simulink model "MODELO_HOGDKING_HUXELY_SBS"  (R2025b)
settings: Solver=ode45  StartTime=0  StopTime=2.5  MaxStep=1e-4  RelTol=1e-3
settings Model: Creator=fabri  LastModifiedBy=fabri

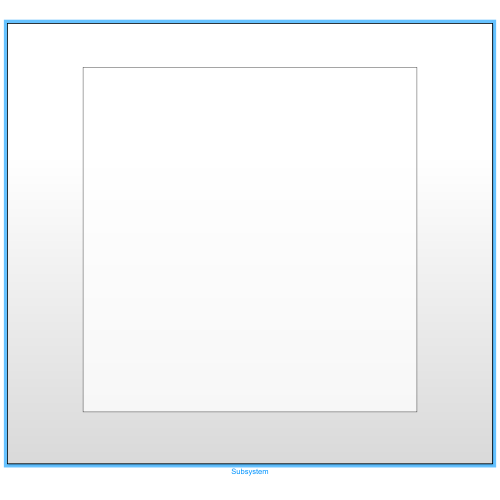
[thumbnail: Simulink's stored preview of the top-level diagram]
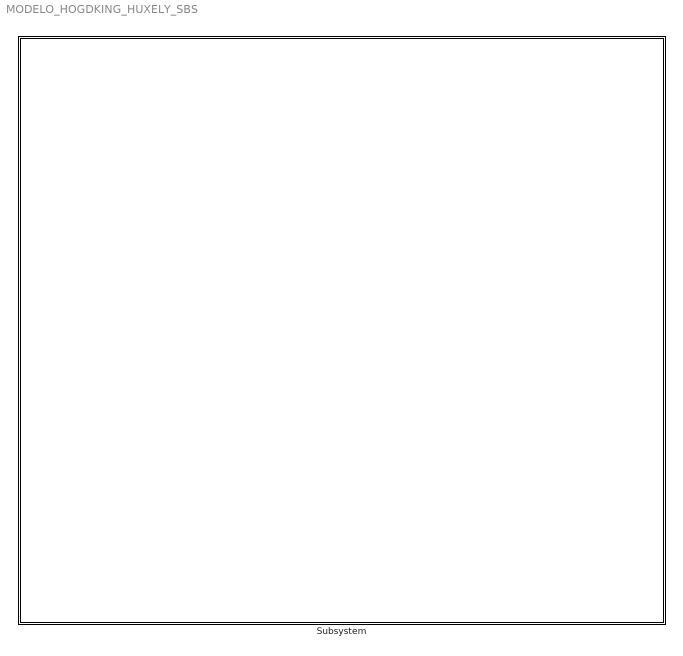
== system MODELO_HOGDKING_HUXELY_SBS ==
  Subsystem : Subsystem

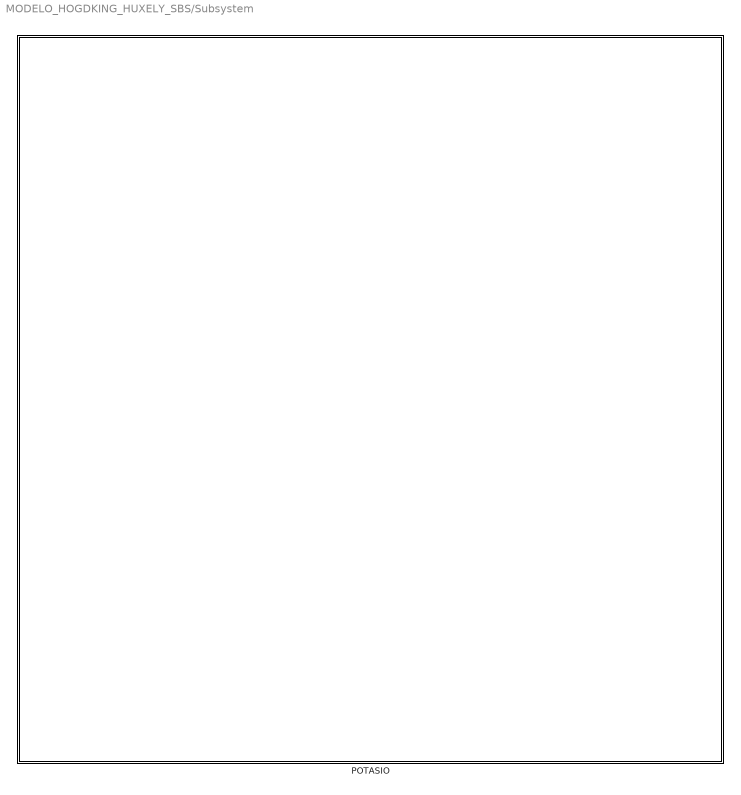
== system MODELO_HOGDKING_HUXELY_SBS/Subsystem ==
  POTASIO : Subsystem

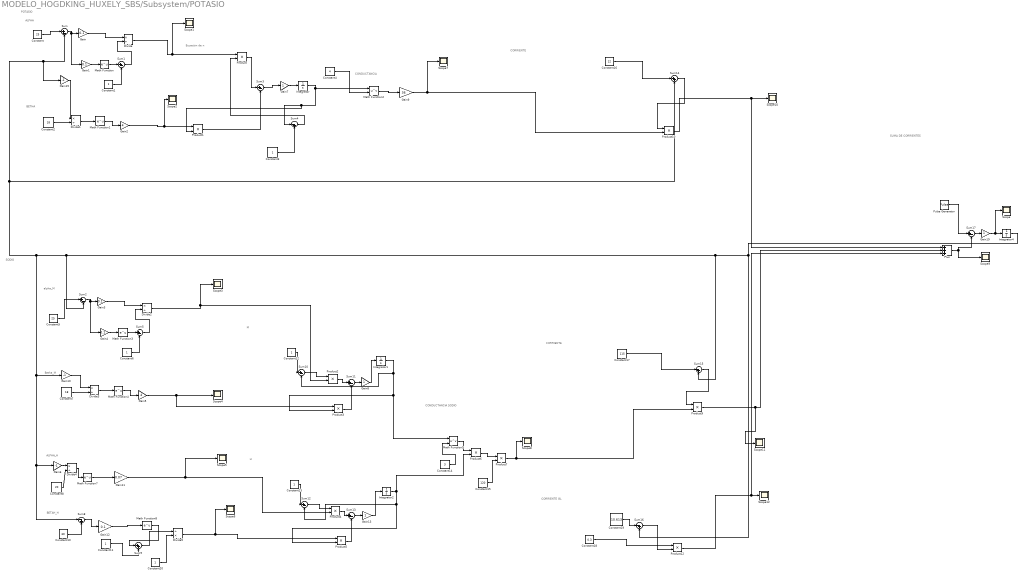
== system MODELO_HOGDKING_HUXELY_SBS/Subsystem/POTASIO ==
  note: CONDUCTANCIA SODIO
  note: M
  note: BETAH_H
  note: CONDUCTANCIA
  note: SODIO
  note: POTASIO
  note: Ecuación de n
  note: BETHA
  note: ALPHA
  note: alpha_M
  note: Betha_M
  note: ALPHA_H
  note: H
  note: CORRIENTE
  note: CORRIENTE
  note: SUMA DE CORRIENTES
  note: CORRIENTE GL
  Constant : Constant  Value=25
  Constant{1,3,6,11..13,20} (7 alike) : Constant
  Constant10 : Constant  Value=30
  Constant14 : Constant  Value=3
  Constant15 : Constant  Value=120
  Constant16 : Constant  Value=12
  Constant17 : Constant  Value=115
  Constant18 : Constant  Value=0.3
  Constant19 : Constant  Value=10.613
  Constant2 : Constant  Value=18
  Constant4 : Constant  Value=4
  Constant5 : Constant  Value=25
  Constant7 : Constant  Value=18
  Constant8 : Constant  Value=20
  Divide{,1..4} (5 alike) : Product  Inputs=*/
  Divide5 : Product  Inputs=/*
  Gain{,1,3..4,12} (5 alike) : Gain  Gain=0.1
  Gain10 : Gain  Gain=-1
  Gain11 : Gain  Gain=0.07
  Gain{7..8,13,19} (4 alike) : Gain
  Gain15 : Gain  Gain=-1
  Gain2 : Gain  Gain=4
  Gain5 : Gain  Gain=4
  Gain6 : Gain  Gain=-1
  Gain9 : Gain  Gain=36
  Integrator : Integrator  InitialCondition=0.317
  Integrator1 : Integrator  InitialCondition=0.05
  Integrator2 : Integrator  InitialCondition=0.6
  Integrator4 : Integrator  InitialCondition=60
  Math Function{,1,3..4,7..8} (6 alike) : Math
  Math Function2 : Math  Operator=pow
  Math Function9 : Math  Operator=pow
  Plus : Sum  Inputs=+++
  Product{,1..7,9..10,12} (11 alike) : Product
  Pulse Generator : DiscretePulseGenerator  PulseType=Time based  Amplitude=35  Period=50  PulseWidth=0.5  PhaseDelay=3
  Scope{,1..12} (13 alike) : Scope
      Scope settings: ActiveDisplayYMinimum=-95.1723618379546  ActiveDisplayYMaximum=59.6779141090574
      Scope1 settings: ActiveDisplayYMinimum=-0.17507037705461403  ActiveDisplayYMaximum=4.8064923190728459
      Scope10 settings: ActiveDisplayYMinimum=-182.23339181248534  ActiveDisplayYMaximum=1699.0889245773781  DataLoggingVariableName=ScopeData10
      Scope11 settings: ActiveDisplayYMinimum=-1  ActiveDisplayYMaximum=1  DataLoggingVariableName=ScopeData11
      Scope12 settings: ActiveDisplayYMinimum=-1  ActiveDisplayYMaximum=1  DataLoggingVariableName=ScopeData12
      Scope2 settings: ActiveDisplayYMinimum=-0.1237591277053367  ActiveDisplayYMaximum=2.0332343992823678  DataLoggingVariableName=ScopeData2
      Scope3 settings: ActiveDisplayYMinimum=-1  ActiveDisplayYMaximum=1  DataLoggingVariableName=ScopeData3
      Scope4 settings: ActiveDisplayYMinimum=-1  ActiveDisplayYMaximum=1  DataLoggingVariableName=ScopeData4
      Scope5 settings: ActiveDisplayYMinimum=-1  ActiveDisplayYMaximum=1  DataLoggingVariableName=ScopeData5
      Scope6 settings: ActiveDisplayYMinimum=-1  ActiveDisplayYMaximum=1  DataLoggingVariableName=ScopeData6
      Scope7 settings: ActiveDisplayYMinimum=-1  ActiveDisplayYMaximum=1  DataLoggingVariableName=ScopeData7
      Scope8 settings: ActiveDisplayYMinimum=-3.1594248054177867  ActiveDisplayYMaximum=28.524823248760089  DataLoggingVariableName=ScopeData8
      Scope9 settings: ActiveDisplayYMinimum=-1  ActiveDisplayYMaximum=1  DataLoggingVariableName=ScopeData9
  Sum{,1..3,5,10..13,17} (10 alike) : Sum  Inputs=|+-
  Sum14 : Sum  Inputs=|++
  Sum{4,8,15..16} (4 alike) : Sum  Inputs=|-+
  Sum9 : Sum  Inputs=|++
  wires:
  Constant/1 -> Sum/1
  Sum1/1 -> Divide/2
  Divide1/1 -> Math Function1/1
  Math Function/1 -> Sum1/1
  Sum/1 -> Gain1/1, Gain/1
  Constant2/1 -> Divide1/2
  Math Function1/1 -> Gain2/1
  Gain1/1 -> Math Function/1
  Constant1/1 -> Sum1/2
  Gain/1 -> Divide/1
  Product/1 -> Sum3/1
  Product1/1 -> Sum3/2
  Sum3/1 -> Gain7/1
  Integrator/1 -> Product1/2, Sum4/1, Math Function2/1
  Constant3/1 -> Sum4/2
  Sum4/1 -> Product/2
  Constant4/1 -> Math Function2/2
  Math Function4/1 -> Gain5/1
  Sum2/1 -> Gain4/1, Gain3/1
  Constant6/1 -> Sum5/2
  Constant7/1 -> Divide3/2
  Gain3/1 -> Divide2/1
  Divide3/1 -> Math Function4/1
  Gain4/1 -> Math Function3/1
  Constant5/1 -> Sum2/1
  Math Function3/1 -> Sum5/1
  Sum5/1 -> Divide2/2
  Math Function2/1 -> Gain9/1
  Math Function7/1 -> Gain11/1
  Constant10/1 -> Sum8/2
  Sum8/1 -> Gain12/1
  Constant11/1 -> Sum9/2
  Integrator1/1 -> Sum10/2, Math Function9/1, Product3/2
  Constant12/1 -> Sum10/1
  Sum10/1 -> Product2/1
  Product2/1 -> Sum11/1
  Product3/1 -> Sum11/2
  Sum11/1 -> Gain8/1
  Sum13/1 -> Gain13/1
  Sum12/1 -> Product4/1
  Divide5/1 -> Scope6/1, Product5/1
  Constant13/1 -> Sum12/1
  Product4/1 -> Sum13/1
  Product5/1 -> Sum13/2
  Integrator2/1 -> Sum12/2, Product5/2, Product6/2
  Constant14/1 -> Math Function9/2
  Math Function9/1 -> Product6/1
  Product6/1 -> Product7/1
  Constant15/1 -> Product7/2
  Product7/1 -> Scope8/1, Product9/2
  Constant16/1 -> Sum14/1
  Sum14/1 -> Product10/1
  Constant17/1 -> Sum15/1
  Constant18/1 -> Product12/1
  Constant19/1 -> Sum16/1
  Sum16/1 -> Product12/2
  Plus/1 -> Sum17/2, Scope9/1
  Constant20/1 -> Divide5/2
  Math Function8/1 -> Sum9/1
  Sum9/1 -> Divide5/1
  Gain12/1 -> Math Function8/1
  Gain9/1 -> Scope7/1, Product10/2
  Sum15/1 -> Product9/1
  Product12/1 -> Plus/3, Scope12/1
  Product10/1 -> Plus/1, Scope10/1
  Pulse Generator/1 -> Sum17/1
  Sum17/1 -> Gain19/1
  Gain7/1 -> Integrator/1
  Gain8/1 -> Integrator1/1
  Gain13/1 -> Integrator2/1
  Divide/1 -> Scope1/1, Product/1
  Divide2/1 -> Scope3/1, Product2/2
  Gain5/1 -> Scope4/1, Product3/1
  Gain19/1 -> Scope/1, Integrator4/1
  Gain15/1 -> Divide1/1
  Gain2/1 -> Scope2/1, Product1/1
  Gain11/1 -> Scope5/1, Product4/2
  Constant8/1 -> Divide4/2
  Gain6/1 -> Divide4/1
  Divide4/1 -> Math Function7/1
  Integrator4/1 -> Sum15/2, Sum2/2, Sum8/1, Gain6/1, Gain10/1, Gain15/1, Sum/2, Sum14/2, Sum16/2
  Gain10/1 -> Divide3/1
  Product9/1 -> Scope11/1, Plus/2
